simulink model "external_entity"  (R2021b)
settings: Solver=FixedStepAuto  StartTime=0.0  StopTime=10.0  RelTol=1e-3
undefined symbols (not defined in the file or in its folder): DiscIntNeverNeededParam, sldvsubsys
libraries: sldvlib x1
settings Model: Creator=marco  LastModifiedBy=angelo
settings ConfigComp: DVMode=PropertyProving  DVTestSuiteOptimization=Auto  DVDetectOutOfBounds=on  DVMaxViolationSteps=5  DVModelReferenceHarness=on

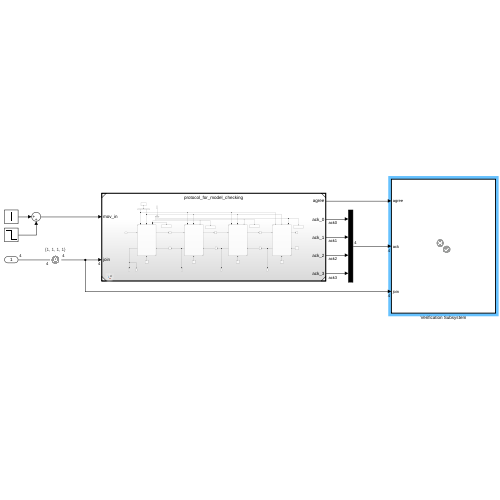
[thumbnail: Simulink's stored preview of the top-level diagram]
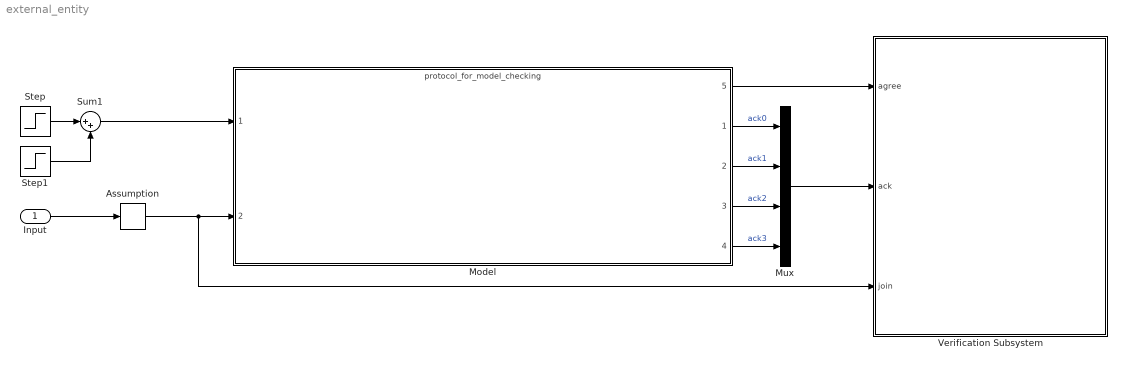
== system external_entity ==
  Input : Inport
  Assumption : sldvlib/Objectives and Constraints/Assumption  enabled=on  customAVTBlockType=Assumption  intervals={1, 1, 1, 1}  initial=off  dispValues=on  outEnabled=on
      settings: AttributesFormatString=%<intervals>  SourceProductBaseCode=SL
  Model : ModelReference  ModelNameDialog=protocol_for_model_checking.slx  SimulationMode=Normal  ModelReferenceVersion=1.33
      settings: PortSchema="{\"entries\":[{\"content\":{\"sides\":[{\"content\":{\"connectorIds\":[\"In1\",\"In2\"]},\"type\":\"ConnectorPlacement.EquallySpacedRectSide\",\"uuid\":\"c0af7f57-5480-49a4-8911-8762eb722174\"},{\"content\":{\"connectorIds\":[\"Out5\",\"Out1\",\"Out2\",\"Out3\",\"Out4\"],\"side\":\"RIGHT\"},\"type\":\"ConnectorPlacement.EquallySpacedRectSide\",\"uuid\":\"6230bb88-e2b9-4468-828b-e08df57f5daf\"},{\"content\":{\"connectorIds\":[],\"side\":\"TOP\"},\"type\":\"ConnectorPlacement.EquallySpacedRectSide\",\"uuid\":\"0c8779a8-0eed-4872-9a95-9fa7713e314c\"}]},\"type\":\"ConnectorPlacement.EquallySpacedConnector\",\"uuid\":\"a0a12abb-5edc-4557-ab0c-1a8aa8a65a2b\"}],\"packageUris\":[\"http://schema.mathworks.com/mf0/Connector/R2020b\"],\"version\":\"1.0\"}"
  Mux : Mux
  Step : Step  Time=0.4  Before=-1  After=0  SampleTime=0.2
  Step1 : Step  Time=0.6  After=-1  SampleTime=0.2
  Sum1 : Sum  Inputs=|++
  Verification Subsystem : Subsystem  Tag=VerificationSubsystem  DisableCoverage=on  LoadFcn=sldvsubsys('check')  TreatAsAtomicUnit=on  SimViewingDevice=on  mask(VerificationSubsystem){}
      mask init:
      | sldvsubsys('maskInit');
      settings: CopyFcn=sldvsubsys('copy');  OpenFcn=open_system(gcb,'force');
      settings: PreSaveFcn=|
      | set_param(gcb,'SimViewingDevice','on');
      | sldvsubsys('check');
      mask Help: helpview(fullfile(docroot,'toolbox','sldv','sldv.map'),'verificationsubsystem')
      mask Display: image(imread('sldvicon_versubsys.png','BackGroundColor',[1 1 1]),'center');
  wires:
  Assumption/1 -> Verification Subsystem/3(join), Model/2
  Input/1 -> Assumption/1
  Model/5 -> Verification Subsystem/1(agree)
  Model/1 -> Mux/1  "ack0"
  Model/2 -> Mux/2  "ack1"
  Model/3 -> Mux/3  "ack2"
  Model/4 -> Mux/4  "ack3"
  Mux/1 -> Verification Subsystem/2(ack)
  Step/1 -> Sum1/1
  Step1/1 -> Sum1/2
  Sum1/1 -> Model/1

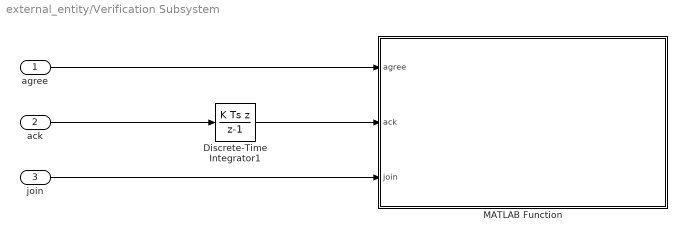
== system external_entity/Verification Subsystem ==
  agree : Inport
  ack : Inport  Port=2
  join : Inport  Port=3
  Discrete-Time Integrator1 : DiscreteIntegrator  IntegratorMethod=Integration: Backward Euler  SampleTime=-1  ICPrevOutput=DiscIntNeverNeededParam  ICPrevScaledInput=DiscIntNeverNeededParam
  MATLAB Function : MATLAB Function  TreatAsAtomicUnit=on
  wires:
  agree/1 -> MATLAB Function/1(agree)
  join/1 -> MATLAB Function/3(join)
  ack/1 -> Discrete-Time Integrator1/1
  Discrete-Time Integrator1/1 -> MATLAB Function/2(ack)

== matlab function external_entity/Verification Subsystem/MATLAB Function ==
  data: agree input; ack input; join input
function validity(agree, ack, join)
    if(agree)
        ack = ack > 0;
        sldv.prove(all(ack == (join & ack)));
    end
end
